simulink model "SCUTERacing_Model"  (R2020a)
settings: Solver=ode23tb  StartTime=0.0  StopTime=60  RelTol=5e-3
model workspace (MAT data in the model file):
  DLCXref = [0 8 9.5 18 34 34.5 45 50 60]
  DLCYref = [0 0 -4.5 -4 -3.75 1.5 0.5 0 0]
  VEH.Mass = 330
  VEH.StaticNormalFrontLoad.FR = 74.25
  VEH.StaticNormalFrontLoad.FL = 74.25
  VEH.StaticNormalRearLoad.RR = 90.75
  VEH.StaticNormalRearLoad.RL = 90.75
  VEH.WheelBase = 1.54
  VEH.FrontAxlePositionfromCG = 0.847
  VEH.RearAxlePositionfromCG = 0.693
  VEH.HeightCG = 0.283
  VEH.FrontalArea = 2.11
  VEH.DragCoefficient = 0.33
  VEH.NumberOfWheelsPerAxle = 2
  VEH.Thread.FR = 1.705
  VEH.Thread.RR = 1.705
  VEH.PitchMomentInertia = 206
  VEH.RollMomentInertia = 206.613792
  VEH.YawMomentInertia = 206.613792
  VEH.SteeringRatio = 5.2
  VEH.TrackWidth = 1.2
  VEH.SprungMass = 290
  VEH.InitialLongPosition = 0
  VEH.InitialLatPosition = 0
  VEH.InitialVertPosition = 0
  VEH.InitialRollAngle = 0
  VEH.InitialPitchAngle = 0
  VEH.InitialYawAngle = 0
  VEH.InitialLongVel = 0
  VEH.InitialLatVel = 0
  VEH.InitialVertVel = 0
  VEH.InitialRollRate = 0
  VEH.InitialPitchRate = 0
  VEH.InitialYawRate = 0
  extRef = 0.01
  mot.max_trq = 135
  mot.max_pwr = 38
  mot.spd = [370 739.166666667 1108.33333333 1477.5 1846.66666667 2215.83333333 2585 2954.16666667 3323.33333333 3692.5 4061.66666667 4430.83333333 4800]
  mot.trq = [135 135 135 135 135 135 130 125 120 90 80 72 65]
  mot.trq_cp = [120 112.169118269 105.297671501 99.2195136541 93.8047673037 88.9504392721 84.5738066939 80.6076640699 76.9968477689 73.6956545886 70.6658970819 90.4670202838 85.9436692696 81.8511135901 78.1306084269 74.7336254518 71.6197243914 68.7549354157]
  mot.mapL.spdindex = [100 200 300 400 500 600 700 800 900 1000 1100 1200 1300 1400 1500 1600 1700 1800 1900 2000 2100 2200 2300 2400 2500 2600 2700 2800 2900 3000 3100 3200 3300 3400 3500 3600 3700 3800 3900 4000 4100 4200 4300 4400 4500 4600 4700 4800]
  mot.mapL.trqindex = [7.5 15 22.5 30 37.5 45 52.5 60 67.5 75 82.5 90 97.5 105 112.5]
  mot.mapL.eff = [23.367031145 28.3093935 27.900833785 23.94351616 23.192960095 18.35774057 20.08454116 17.944414665 15.71176136 14.08332132 13.191387315 11.66605693 ... (720 elements, 15x48)]
  mot.mapR.spdindex = [100 200 300 400 500 600 700 800 900 1000 1100 1200 1300 1400 1500 1600 1700 1800 1900 2000 2100 2200 2300 2400 2500 2600 2700 2800 2900 3000 3100 3200 3300 3400 3500 3600 3700 3800 3900 4000 4100 4200 4300 4400 4500 4600 4700 4800]
  mot.mapR.trqindex = [7.5 15 22.5 30 37.5 45 52.5 60 67.5 75 82.5 90 97.5 105 112.5]
  mot.mapR.eff = [28.48167539 36.0807345 35.29712042 34.7163836 33.02727304 31.53442549 31.60094145 28.55014096 26.94374363 27.02005929 24.78971019 24.19758491 ... (720 elements, 15x48)]
undefined symbols (not defined in the file or in its folder): Batt, h, Right
libraries: simulink x6, vehdynlibscenariocommon x4, sim3dlib x2, vehdynlibdriver x1, autolibshared x1, vehdynlibviscommon x1
(part 1 of 2)
settings Model: SimulationMode=accelerator  Creator=Administrator  LastModifiedBy=Administrator
settings SolverCC: ZeroCrossAlgorithm=Adaptive
settings DataIOCC: DSMLogging=off
settings DebuggingCC: IgnoredZcDiagnostic=none

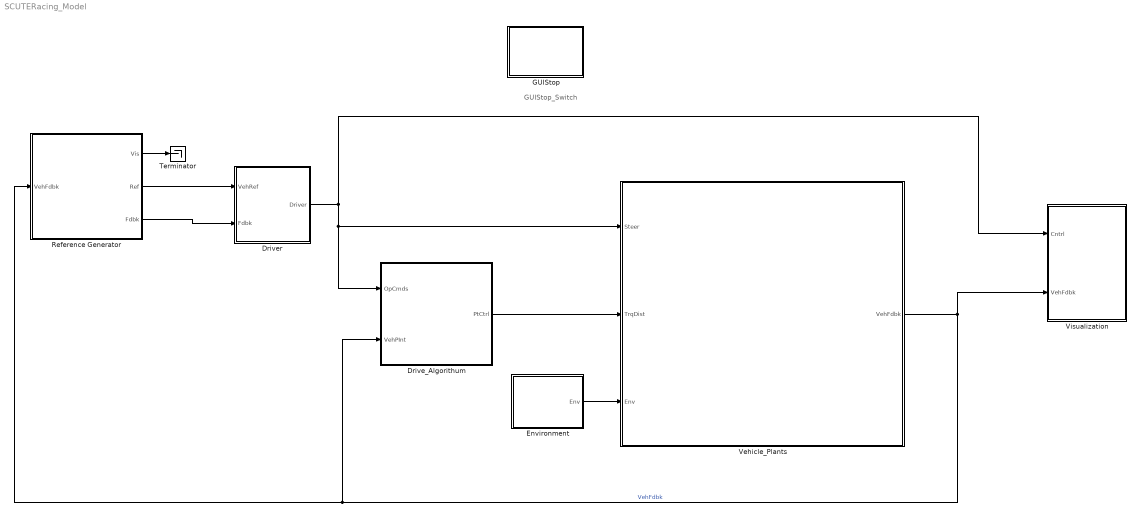
== system SCUTERacing_Model ==
  note: GUIStop_Switch
  Drive_Algorithum : Subsystem
      mask Display: image("Model_Pictures/SystemControllers.png")
  Driver : Subsystem
      mask Display: image("Model_Pictures/LongitudinalDriver.png")
  Environment : Subsystem
  GUIStop : Subsystem
  Reference Generator : Subsystem  Variant=on  VariantControl=Variant1
  Terminator : Terminator
  Vehicle_Plants : Subsystem
      mask Display: image("Model_Pictures/PassengerVehicle.png")
  Visualization : Subsystem
  wires:
  Reference Generator/1(" Vis") -> Terminator/1
  Reference Generator/2(" Ref") -> Driver/1(VehRef)
  Reference Generator/3(" Fdbk") -> Driver/2(Fdbk)
  Drive_Algorithum/1(PtCtrl) -> Vehicle_Plants/2(TrqDist)
  Vehicle_Plants/1(VehFdbk) -> Visualization/2(VehFdbk), Reference Generator/1("VehFdbk "), Drive_Algorithum/2(VehPInt)  "VehFdbk"
  Driver/1(Driver) -> Drive_Algorithum/1(OpCmds), Vehicle_Plants/1(Steer), Visualization/1(Cntrl)
  Environment/1(Env) -> Vehicle_Plants/3(Env)

== system SCUTERacing_Model/Drive_Algorithum ==
  OpCmds : Inport
  VehPInt : Inport  Port=2
  Algorithum : Subsystem
  outport_Module : Subsystem
  PtCtrl : Outport
  wires:
  Algorithum/1(BrakeCmd) -> outport_Module/1(BrakeCmd)
  VehPInt/1 -> Algorithum/2(VehPInt)
  Algorithum/2(MotCmd_L) -> outport_Module/2(MotCmd_L)
  Algorithum/3(MotCmd_R) -> outport_Module/3(MotCmd_R)
  outport_Module/1(OpCmd) -> PtCtrl/1
  OpCmds/1 -> Algorithum/1(OpCmds)

== system SCUTERacing_Model/Driver ==
  VehRef : Inport
  Fdbk : Inport  Port=2
  Bus Creator : BusCreator  Inputs=3
  Bus Selector : BusSelector  OutputSignals=Chassis.xdot,Chassis.Y,Chassis.ydot,Chassis.psi,Chassis.r
  Bus Selector1 : BusSelector  OutputSignals=LngRef,LtrlRef,AccelZero
  Constant : Constant  Value=0
  Dead Zone : DeadZone  ZeroCross=off  SaturateOnIntegerOverflow=on
  Dead Zone1 : DeadZone  LowerValue=-1e-2  UpperValue=1e-2  ZeroCross=off  SaturateOnIntegerOverflow=on
  Ground : Ground
  Predictive Driver : vehdynlibdriver/Predictive Driver  extAccelOvr=off  extDecelOvr=off  extAccelHld=off  extDecelHld=off  extAccelZero=off  extDecelZero=off  extSteerOvr=off  extSteerHld=off  extSteerZero=off  cntrlType=PI  shftType=None  velUnits=m/s  gearOut=off  steerOut=off  Kp=10  Ki=5  Kff=.1  Kg=0  VehVelVec=[0 100]  KffVec=[.1 .1]  KpVec=[10 10]  KiVec=[5 5]  KgVec=[0 0]  vnom=35  Kaw=1  tauerr=.01  a=VEH.FrontAxlePositionfromCG  b=VEH.RearAxlePositionfromCG  m=VEH.Mass  I=VEH.YawMomentInertia  Cy_f=11459  Cy_r=11459  theta=30*pi/180  Ksteer=18  tau=0.03  L=1.0  Kpt=3000  aR=200  bR=2.5  cR=.5  g=9.81  GearInit=0  tShift=.1  pdlVec=[0.1 0.4 0.5 0.9]  upShftTbl=[-1 12.9375 26.4375 39.9375 51.18749999999999 62.4375 72.84375 83.25;-1 16.3125 29.8125 43.3125 54.5624 65.8125 76.78125 87.75;-1 19.6875 33.1875 46.68749999999999 57.9375 69.1875 80.71875 92.25;-1 33 52.5 77.25 100.5 138.75 161.875 185]  dwnShftTbl=[-1 12.9375 26.4375 39.9375 51.18749999999999 62.4375 72.84375 83.25;-1 16.3125 29.8125 43.3125 54.5624 65.8125 76.78125 87.75;-1 19.6875 33.1875 46.68749999999999 57.9375 69.1875 80.71875 92.25;-1 33 52.5 77.25 100.5 138.75 161.875 185]  tClutch=.5  tRev=.5  tPark=120  aMode=2  UpGearVec="[0  1  2  3  4  5  6  7]"  DownGearVec="[1  2  3  4  5  6  7  8]"
      settings: SourceProductBaseCode=VE
  Switch : Switch  Criteria=u2 > Threshold
  Terminator1 : Terminator
  Wheel Angle Limit * Steer Ratio : Gain  Gain=20*pi/180*5.2
  Driver : Outport  VectorParamsAs1DForOutWhenUnconnected=off
  wires:
  Fdbk/1 -> Bus Selector/1
  Bus Creator/1 -> Driver/1
  Bus Selector1/1 -> Predictive Driver/1  "<LngRef>"
  Bus Selector/3 -> Predictive Driver/6  "<ydot>"
  Bus Selector/4 -> Predictive Driver/7  "<psi>"
  Switch/1 -> Bus Creator/2  "Accel"
  Bus Selector/1 -> Dead Zone/1  "<xdot>"
  Predictive Driver/3 -> Switch/3  "AccelCmd"
  Bus Selector1/2 -> Predictive Driver/2  "<LtrlRef>"
  Dead Zone/1 -> Predictive Driver/4
  Bus Selector/2 -> Predictive Driver/5  "<Y>"
  Dead Zone1/1 -> Wheel Angle Limit * Steer Ratio/1
  Predictive Driver/4 -> Bus Creator/3  "Brake"
  Wheel Angle Limit * Steer Ratio/1 -> Bus Creator/1  "Steer"
  Predictive Driver/1 -> Terminator1/1
  Bus Selector1/3 -> Switch/2  "<AccelZero>"
  Bus Selector/5 -> Predictive Driver/8  "<r>"
  Constant/1 -> Switch/1
  Ground/1 -> Predictive Driver/3
  VehRef/1 -> Bus Selector1/1
  Predictive Driver/2 -> Dead Zone1/1  "SteerCmd"

== system SCUTERacing_Model/Environment ==
  note: 注释：
      | 1）输入：
      | 1.Temp:环境温度
      | 2.Wind:模拟风速（x,y,z三个坐标）
      | 3.Gnd: a.G
      | b. friction:摩擦力（FL：前左轮；FR：前右轮；RL：后左轮；FL:后右轮）
      |
      | 2）输出：
      | 环境条件 Env ：
      | Temp：温度
      | Wind：风向
      | Gnd：地面参数
  Bus Creator : BusCreator  Inputs=4
  Bus Creator1 : BusCreator  Inputs=3
  Bus Creator2 : BusCreator  Inputs=4
  Bus Creator3 : BusCreator  Inputs=2
  Constant1 : Constant  Value=zeros(4,1)
  Constant3 : Constant  Value=0
  Constant4 : Constant  Value=0
  Constant5 : Constant  Value=0
  Constant6 : Constant  Value=300
  Demux : Demux
  Demux1 : Demux
  Friction : Constant  Value=ones(4,1).*1
  Vector Concatenate : Concatenate  NumInputs=3
  Env : Outport  VectorParamsAs1DForOutWhenUnconnected=off
  wires:
  Friction/1 -> Demux1/1
  Demux1/4 -> Bus Creator2/4  "mu_RR"
  Demux1/3 -> Bus Creator2/3  "mu_RL"
  Demux/1 -> Bus Creator/1  "G_FL_z"
  Vector Concatenate/1 -> Bus Creator1/2  "Wind"
  Demux1/1 -> Bus Creator2/1  "mu_FL"
  Constant1/1 -> Demux/1
  Bus Creator1/1 -> Env/1
  Bus Creator3/1 -> Bus Creator1/3  "Gnd"
  Demux1/2 -> Bus Creator2/2  "mu_FR"
  Constant6/1 -> Bus Creator1/1  "Temp"
  Demux/4 -> Bus Creator/4  "G_RR_z"
  Constant4/1 -> Vector Concatenate/2  "Y"
  Demux/2 -> Bus Creator/2  "G_FR_z"
  Demux/3 -> Bus Creator/3  "G_RL_z"
  Constant3/1 -> Vector Concatenate/1  "X"
  Constant5/1 -> Vector Concatenate/3  "Z"
  Bus Creator/1 -> Bus Creator3/1  "z"
  Bus Creator2/1 -> Bus Creator3/2  "mu"

== system SCUTERacing_Model/GUIStop ==
  S-Function : S-Function  FunctionName=StopFlag  SFunctionDeploymentMode=off  EnableBusSupport=off
  Stop Simulation : Stop
  wires:
  S-Function/1 -> Stop Simulation/1

== system SCUTERacing_Model/Reference Generator ==
  "VehFdbk " : Inport
  Constant Radius : Subsystem  VariantControl=RG==4  mask{t_start=0, xdot_r=120, xdotUnit=mph, R=22.5, turnDirMask=Right, ay_max=0.5, ay_stop=off, Parameter6=2}
      mask prompts: t_start "Maneuver start time, t_start [s]:"; xdot_r "Longitudinal velocity reference, xdot_r:"; xdotUnit "Longitudinal velocity reference units, xdotUnit []:"; R "Radius value, R [m]:"; turnDirMask "Turn direction"; ay_max "Lateral acceleration absolute threshold, ay_max [g]:"; ay_stop "Stop simulation at lateral acceleration threshold"
      mask TypeOptions xdotUnit: Longitudinal Velocity Reference/Input Units/Unit
      mask TypeOptions R: Constant Radius/Value
      mask TypeOptions turnDirMask: Constant Radius/turnDirMask
  Increasing Steer : Subsystem  VariantControl=RG==1
  Longitual_increasing : Subsystem  VariantControl=RG==0
  RealRunData : Subsystem  VariantControl=RG==5
  Sine with Dwell : Subsystem  VariantControl=RG==3
  Swept Sine : Subsystem  VariantControl=RG==2
  " Vis" : Outport  VectorParamsAs1DForOutWhenUnconnected=off
  " Ref" : Outport  Port=2  VectorParamsAs1DForOutWhenUnconnected=off
  " Fdbk" : Outport  Port=3  VectorParamsAs1DForOutWhenUnconnected=off

== system SCUTERacing_Model/Vehicle_Plants ==
  Steer : Inport
  TrqDist : Inport  Port=2
  Env : Inport  Port=3
  Bus Creator : BusCreator  Inputs=6
  Elect_Plant : Subsystem
  Steer_Sys : Subsystem
  Vehicle_Body : Subsystem
  VehFdbk : Outport
  wires:
  [MotSpd_L] -> Elect_Plant/5(Veh_L)
  Env/1 -> Elect_Plant/3(Env), Vehicle_Body/1(Env)
  Elect_Plant/1(ElecFdbk) -> Bus Creator/1, [ElecFdbk]  "ElecFdbk"
  [MotSpd_R] -> Elect_Plant/4(Veh_R)
  Vehicle_Body/3(MotSpd_L) -> Bus Creator/5, [MotSpd_L]  "MotSpd_L"
  Steer_Sys/1(DriveLine) -> Bus Creator/2, [DriveLine]  "DriveLine"
  Vehicle_Body/2(Wheels) -> Bus Creator/4, [Wheels]  "Wheels"
  Vehicle_Body/4(MotSpd_R) -> Bus Creator/6, [MotSpd_R]  "MotSpd_R"
  TrqDist/1 -> Elect_Plant/2(Ctrl_L), Steer_Sys/1(Contrl), Elect_Plant/1(Ctrl_R)
  Vehicle_Body/1(Chassis) -> Bus Creator/3  "Chassis"
  [DriveLine] -> Vehicle_Body/2(DriveLine)
  [ElecFdbk] -> Steer_Sys/3(ElecFdbk)
  [Wheels] -> Steer_Sys/4(Wheels)
  Steer/1 -> Steer_Sys/2(Steer)
  Bus Creator/1 -> VehFdbk/1

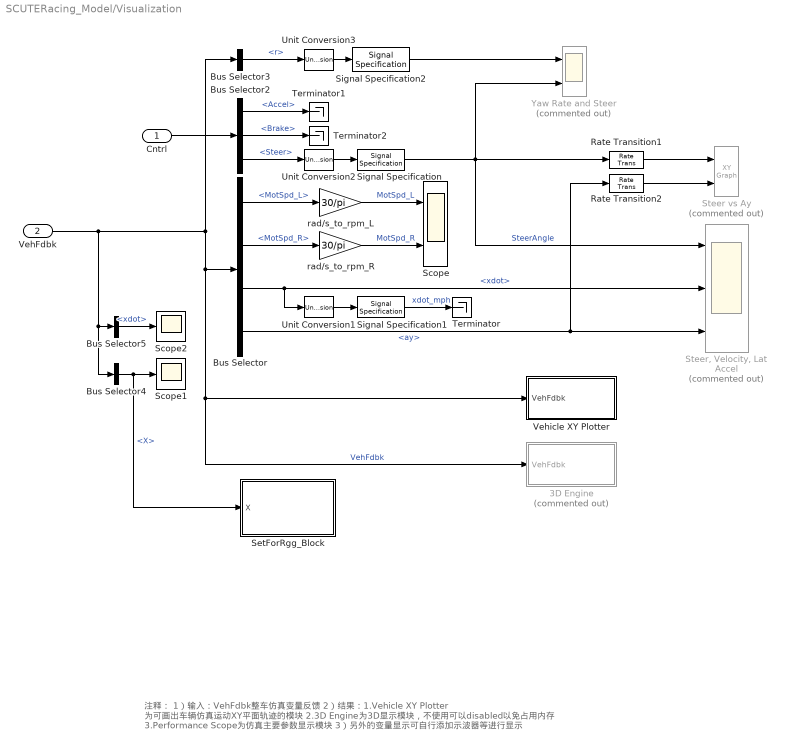
== system SCUTERacing_Model/Visualization ==
  note: 注释：
      | 1）输入：VehFdbk整车仿真变量反馈
      | 2）结果：1.Vehicle XY Plotter 为可画出车辆仿真运动XY平面轨迹的模块
      | 2.3D Engine为3D显示模块，不使用可以disabled以免占用内存
      | 3.Performance Scope为仿真主要参数显示模块
      | 3）另外的变量显示可自行添加示波器等进行显示
  Cntrl : Inport
  VehFdbk : Inport  Port=2
  3D Engine : Subsystem  Commented=on  Variant=on  VariantControlMode=Label  LabelModeActiveChoice=0  mask(3D Engine){engine3D=Disabled, SceneDesc=Straight road, dt3D=.03}
      mask prompts: engine3D "3D Engine"; SceneDesc "Scene Description:"; dt3D "Engine frame rate, dt3D [s]:"
      mask help: This subsystem contains the interface blocks which permit the display of the vehicle in 3D virtual environment. Enable it to view the simulation progress, disable it to inhibit the display.
      mask init:
      | switch get_param(gcb,'engine3D')
      |     case 'Disabled'
      |         set_param(gcb,'OverrideUsingVariant','0')
      |     case 'Enabled'
      |        set_param(gcb,'OverrideUsingVariant','1')
      |     otherwise
      |        set_param(gcb,'OverrideUsingVariant','0')
      | end
      settings: AttributesFormatString=%<engine3D>
      mask Help: eval('vdynblkshelp(''vdynblksscenecameraray'')');
      mask TypeOptions engine3D: Enabled | Disabled
      mask Callback engine3D:
      | switch get_param(gcb,'engine3D')
      |     case 'Disabled'
      |         set_param(gcb,'OverrideUsingVariant','0')
      |     case 'Enabled'
      |        set_param(gcb,'OverrideUsingVariant','1')
      |     otherwise
      |        set_param(gcb,'OverrideUsingVariant','0')
      | end
      mask TypeOptions SceneDesc:
      | 3D Engine/Simulation 3D Engine
      | 1/SceneDesc
      mask Display: disp('3D Engine')
  Bus Selector : BusSelector  OutputSignals=MotSpd_L,MotSpd_R,Chassis.xdot,Chassis.ay
  Bus Selector2 : BusSelector  OutputSignals=Accel,Brake,Steer
  Bus Selector3 : BusSelector  OutputSignals=Chassis.r
  Bus Selector4 : BusSelector  OutputSignals=Chassis.X
  Bus Selector5 : BusSelector  OutputSignals=Chassis.xdot
  Rate Transition1 : RateTransition  OutPortSampleTime=.1
  Rate Transition2 : RateTransition  OutPortSampleTime=.1
  Scope : Scope  NumInputPorts=2
  Scope1 : Scope
  Scope2 : Scope
  SetForRgg_Block : Subsystem
  Signal Specification : SignalSpecification  Unit=deg
  Signal Specification1 : SignalSpecification  Unit=mph
  Signal Specification2 : SignalSpecification  Unit=deg/s
  Steer vs Ay : simulink/Sinks/XY Graph  Commented=on  xmin=-300  xmax=300  ymin=-1.5  ymax=1.5  st=.1
  "Steer, Velocity, Lat Accel" : Scope  Commented=on  NumInputPorts=3
  Terminator : Terminator
  Terminator1 : Terminator
  Terminator2 : Terminator
  Unit Conversion1 : UnitConversion
  Unit Conversion2 : UnitConversion
  Unit Conversion3 : UnitConversion
  Vehicle XY Plotter : Subsystem  mask(Vehicle XY Plotter){a=VEH.FrontAxlePositionfromCG, b=VEH.RearAxlePositionfromCG, w=VEH.TrackWidth, bufferSize=1024, pltDT=.1}
      mask prompts: a "Distance to front axle from CG, a [m]:"; b "Distance to rear axle from CG, b [m]:"; w "Track width, w [m]:"; bufferSize "Path buffer sampe size, bufferSize []:"; pltDT "Plot update rate, pltDT [s]:"
      mask help: This block will display a MATLAB figure which indicates the vehicle path, current position and heading velocity.
      mask TypeOptions a: Vehicle XY Plotter/a
      mask TypeOptions b: Vehicle XY Plotter/b
      mask TypeOptions w: Vehicle XY Plotter/w
      mask TypeOptions bufferSize: Vehicle XY Plotter/bufferSize
  Yaw Rate and Steer : Scope  Commented=on  NumInputPorts=2
  rad/s_to_rpm_L : Gain  Gain=30/pi
  rad/s_to_rpm_R : Gain  Gain=30/pi
  wires:
  Unit Conversion2/1 -> Signal Specification/1
  Signal Specification/1 -> Yaw Rate and Steer/2, Rate Transition1/1, "Steer, Velocity, Lat Accel"/1  "SteerAngle"
  Bus Selector2/1 -> Terminator1/1  "<Accel>"
  Bus Selector3/1 -> Unit Conversion3/1  "<r>"
  Signal Specification2/1 -> Yaw Rate and Steer/1
  Cntrl/1 -> Bus Selector2/1
  Rate Transition2/1 -> Steer vs Ay/2
  Rate Transition1/1 -> Steer vs Ay/1
  rad/s_to_rpm_L/1 -> Scope/1  "MotSpd_L"
  Bus Selector4/1 -> SetForRgg_Block/1(X), Scope1/1  "<X>"
  Bus Selector/2 -> rad/s_to_rpm_R/1  "<MotSpd_R>"
  Bus Selector/1 -> rad/s_to_rpm_L/1  "<MotSpd_L>"
  Bus Selector2/3 -> Unit Conversion2/1  "<Steer>"
  Unit Conversion1/1 -> Signal Specification1/1
  VehFdbk/1 -> Bus Selector5/1, Bus Selector4/1, Bus Selector/1, Vehicle XY Plotter/1(VehFdbk), 3D Engine/1(VehFdbk), Bus Selector3/1  "VehFdbk"
  Bus Selector2/2 -> Terminator2/1  "<Brake>"
  Unit Conversion3/1 -> Signal Specification2/1
  Bus Selector5/1 -> Scope2/1  "<xdot>"
  Signal Specification1/1 -> Terminator/1  "xdot_mph"
  Bus Selector/3 -> Unit Conversion1/1, "Steer, Velocity, Lat Accel"/2  "<xdot>"
  rad/s_to_rpm_R/1 -> Scope/2  "MotSpd_R"
  Bus Selector/4 -> Rate Transition2/1, "Steer, Velocity, Lat Accel"/3  "<ay>"

== system SCUTERacing_Model/Drive_Algorithum/Algorithum ==
  OpCmds : Inport
  VehPInt : Inport  Port=2
  Algorithum_VariantModel : Subsystem  Variant=on
  Mux : Mux
  "Power Management " : Subsystem
  Subsystem : Subsystem
  inportModule : Subsystem
  BrakeCmd : Outport
  MotCmd_L : Outport  Port=2
  MotCmd_R : Outport  Port=3
  wires:
  Mux/1 -> BrakeCmd/1
  OpCmds/1 -> inportModule/1(OpCmds)
  VehPInt/1 -> inportModule/2(VehPInt)
  inportModule/1(AccCmd) -> Subsystem/2(AccCmd), Algorithum_VariantModel/1(AccCmd)
  inportModule/10(WhlAng) -> Algorithum_VariantModel/10(WhlAng)
  inportModule/11(Spd) -> Algorithum_VariantModel/11(Spd)
  inportModule/8(Steer) -> Algorithum_VariantModel/8(Steer)
  inportModule/9(YawRate) -> Algorithum_VariantModel/9(YawRate)
  inportModule/2(MotSpd_L) -> [MotSpd_L], Subsystem/3(MotSpd_L), Algorithum_VariantModel/2(MotSpd_L)
  inportModule/3(MotSpd_R) -> [MotSpd_R], Subsystem/1(MotSpd_R), Algorithum_VariantModel/3(MotSpd_R)
  inportModule/4(VehSpd(km/h)) -> Algorithum_VariantModel/4(VehSpd)
  inportModule/5(DecCmd) -> Algorithum_VariantModel/5(DecCmd)
  inportModule/6(MotPwr_L) -> Algorithum_VariantModel/6(MotPwr_L)
  inportModule/7(MotPwr_R) -> Algorithum_VariantModel/7(MotPwr_R)
  inportModule/12(BattSOC) -> Algorithum_VariantModel/12(BattSOC)
  Subsystem/1(MotTrqCmd_L) -> Algorithum_VariantModel/13(MotTrqCmd_L)
  Subsystem/2(MotTrqCmd_R) -> Algorithum_VariantModel/14(MotTrqCmd_R)
  Algorithum_VariantModel/3(Fric_Brake) -> Mux/4, Mux/3, Mux/2, Mux/1
  Algorithum_VariantModel/1(Final_MotTrqReq_L) -> "Power Management "/1(MotTrqReq_L)
  Algorithum_VariantModel/2(Final_MotTrqReq_R) -> "Power Management "/2(MotTrqReq_R)
  inportModule/13(BattVolt) -> [BattVolt]
  [MotSpd_R] -> "Power Management "/4(MotSpd_R)
  [MotSpd_L] -> "Power Management "/3(MotSpd_L)
  [BattVolt] -> "Power Management "/5(BattV)
  "Power Management "/2(MotTrqReqAllow_R) -> MotCmd_R/1
  "Power Management "/1(MotTrqReqAllow_L) -> MotCmd_L/1

== system SCUTERacing_Model/Drive_Algorithum/outport_Module ==
  BrakeCmd : Inport
  MotCmd_L : Inport  Port=2
  MotCmd_R : Inport  Port=3
  Bus Creator : BusCreator  Inputs=3
  Memory : Memory
  Rate Transition : RateTransition  Deterministic=off
  Rate Transition1 : RateTransition  Deterministic=off
  Rate Transition2 : RateTransition  Deterministic=off
  OpCmd : Outport
  wires:
  BrakeCmd/1 -> Rate Transition/1
  MotCmd_L/1 -> Rate Transition1/1
  MotCmd_R/1 -> Rate Transition2/1
  Rate Transition/1 -> Memory/1
  Rate Transition1/1 -> Bus Creator/2  "MotCmd_L"
  Rate Transition2/1 -> Bus Creator/3  "MotCmd_R"
  Bus Creator/1 -> OpCmd/1
  Memory/1 -> Bus Creator/1  "BrakeCmd"

== system SCUTERacing_Model/Reference Generator/Constant Radius ==
  "VehFdbk " : Inport
  Bus Assignment : BusAssignment  AssignedSignals=Chassis.Y
  Bus Creator : BusCreator  Inputs=3
  Bus Creator1 : BusCreator  Inputs=5
  Bus Selector1 : BusSelector  OutputSignals=Chassis.ay
  Bus Selector2 : BusSelector  OutputSignals=Chassis.X,Chassis.Y,Chassis.psi,Chassis.Z
  Constant : Constant  Value=0
  Constant Radius : Subsystem  mask{Value=R, turnDirMask=Right}
      mask prompts: Value "Simulink:blkprm_prompts:ConstConstValue"; turnDirMask "Turn direction"
      mask TypeOptions Value: R/Value
      mask TypeOptions turnDirMask: Left | Right
      mask DialogControl Value Prompt: Constant value:
  Constant1 : Constant  Value=0  OutDataTypeStr=boolean
  Constant2 : Constant  Value=0
  Constant3 : Constant  Value=0  OutDataTypeStr=boolean
  Longitudinal Velocity Reference : Subsystem
  Signal Copy : SignalConversion  OverrideOpt=off
  Signal Specification : SignalSpecification  Unit=m
  ay Stop : vehdynlibscenariocommon/Slowly Increasing Steer/ay Stop  SystemSampleTime=-1  Latency=0  AutoFrameSizeCalculation=off
      settings: SourceProductBaseCode=VE
  " Vis" : Outport  VectorParamsAs1DForOutWhenUnconnected=off
  " Ref" : Outport  Port=2  VectorParamsAs1DForOutWhenUnconnected=off
  " Fdbk" : Outport  Port=3  VectorParamsAs1DForOutWhenUnconnected=off
  wires:
  Constant3/1 -> Bus Creator1/3  "EnblSteerCmd"
  Constant2/1 -> Bus Creator1/4  "SteerOvrCmd"
  Longitudinal Velocity Reference/1(xdot) -> Bus Creator1/1  "LngRef"
  Signal Specification/1 -> Bus Creator1/2  "LtrlRef"
  Bus Creator1/1 -> " Ref"/1
  Constant1/1 -> Bus Creator1/5  "AccelZero"
  Constant/1 -> Signal Specification/1
  Constant Radius/1(yRef) -> Bus Assignment/2  "LatRef"
  Bus Assignment/1 -> " Fdbk"/1
  Signal Copy/1 -> Bus Creator/3  "ZRef"
  Bus Creator/1 -> " Vis"/1
  Bus Selector2/4 -> Signal Copy/1  "<Z>"
  Constant Radius/3(YRef) -> Bus Creator/2  "YRef"
  "VehFdbk "/1 -> Bus Selector2/1, Bus Assignment/1, Bus Selector1/1
  Bus Selector2/2 -> Constant Radius/2(YVeh)  "<Y>"
  Bus Selector2/3 -> Constant Radius/3(psiVeh)  "<psi>"
  Bus Selector2/1 -> Constant Radius/1(XVeh)  "<X>"
  Constant Radius/2(XRef) -> Bus Creator/1  "XRef"
  Bus Selector1/1 -> ay Stop/1  "<ay>"

== system SCUTERacing_Model/Reference Generator/Increasing Steer ==
  "VehFdbk " : Inport
  Bus Creator : BusCreator  Inputs=3
  Ground : Ground
  Ground1 : Ground
  Ground2 : Ground
  Increasing Steer : vehdynlibscenariocommon/Slowly Increasing Steer  VariantControl=1  t_start=0  xdot_r=35  xdotUnit=mph  omega_hw=13.5  theta_max=90  t_stop=60  ay_max=0.5  ay_stop=on  aMode=2
      settings: SourceProductBaseCode=VE
  " Vis" : Outport  VectorParamsAs1DForOutWhenUnconnected=off
  " Ref" : Outport  Port=2  VectorParamsAs1DForOutWhenUnconnected=off
  " Fdbk" : Outport  Port=3  VectorParamsAs1DForOutWhenUnconnected=off
  wires:
  Ground/1 -> Bus Creator/1  "XRef"
  Ground1/1 -> Bus Creator/2  "YRef"
  Ground2/1 -> Bus Creator/3  "ZRef"
  Increasing Steer/1 -> " Ref"/1  "LtrlRef"
  Bus Creator/1 -> " Vis"/1
  "VehFdbk "/1 -> Increasing Steer/1, " Fdbk"/1

== system SCUTERacing_Model/Reference Generator/Longitual_increasing ==
  "VehFdbk " : Inport
  Bus Creator : BusCreator  Inputs=3
  Ground : Ground
  Ground1 : Ground
  Ground2 : Ground
  Ramp : simulink/Sources/Ramp  slope=100  start=0  InitialOutput=0  VectorParams1D=off
  Saturation : Saturate  UpperLimit=80
      settings: LockScale=on
  Signal Specification1 : SignalSpecification  Unit=m/s
  Signal Specification2 : SignalSpecification  Unit=mph
  Unit Conversion1 : UnitConversion
  " Vis" : Outport
  " Ref" : Outport  Port=2
  " Fdbk" : Outport  Port=3
  wires:
  "VehFdbk "/1 -> " Fdbk"/1
  Ground/1 -> " Vis"/1
  Ramp/1 -> Saturation/1
  Unit Conversion1/1 -> Signal Specification1/1
  Bus Creator/1 -> " Ref"/1
  Signal Specification1/1 -> Bus Creator/1  "LngRef"
  Ground1/1 -> Bus Creator/2  "LtrlRef"
  Ground2/1 -> Bus Creator/3  "AccelZero"
  Saturation/1 -> Signal Specification2/1
  Signal Specification2/1 -> Unit Conversion1/1  "Km/h"

== system SCUTERacing_Model/Reference Generator/RealRunData ==
  "VehFdbk " : Inport
  Bus Creator : BusCreator  Inputs=3
  Drive Cycle Source : autolibshared/Drive Cycle Source  cycleVar=.mat, .xls, .xlsx or .txt file  fileVar=C:\Users\Administrator\Desktop\新建文件夹 (3)\Scutracing\SCUTRacing\Eracing2020\SCUTRacing_EF20SimulinkProject\mFile\xdotref.mat  tfinal="2273  seconds"  cycleRepeat=off  outAccPort=off  outGearPort=off  gearList=No gear data  t_wot1=5  xdot_woto=0  xdot_wot1=30  t_wot2=20  xdot_wot2=0  t_wotend=30  srcUnit=km/h  outUnit=mph  srcAccUnit=m/s/s  outAccUnit=m/s^2  dt=0  aMode=1  faultOption=off  velBnd=2  velBndUnit=mph  inUnit=m/s  timeBnd=1  failOption=off  stopSim=off  maxFaultCnt=10  maxFaultTime=2  maxTotFaultTime=15  traceOption=off  dtTrace=1  traceWindow=10  lastDCname=Custom Data Set  lastOutUnit=mph  lastDT=0  lastTB=1  lastSB=2  forceCalcBound=off
      settings: AttributesFormatString=耐久跑动3圈数据 (%<tfinal>)  SourceProductBaseCode=PW
  Ground : Ground
  Ground1 : Ground
  Ground2 : Ground
  SetForRgg_Block2 : Subsystem  Commented=on
  " Vis" : Outport
  " Ref" : Outport  Port=2
  " Fdbk" : Outport  Port=3
  wires:
  "VehFdbk "/1 -> " Fdbk"/1
  Ground/1 -> " Vis"/1
  Bus Creator/1 -> " Ref"/1
  Drive Cycle Source/1 -> SetForRgg_Block2/1(LngRef), Bus Creator/1  "LngRef"
  Ground1/1 -> Bus Creator/2  "LtrlRef"
  Ground2/1 -> Bus Creator/3  "AccelZero"

== system SCUTERacing_Model/Reference Generator/Sine with Dwell ==
  "VehFdbk " : Inport
  Bus Creator : BusCreator  Inputs=3
  Ground : Ground
  Ground1 : Ground
  Ground2 : Ground
  Sine With Dwell : vehdynlibscenariocommon/Sine With Dwell  VariantControl=3  t_start=0  xdot_r=30  xdotUnit=mph  steerF=7  steerA=90  tdwell=0.5  steerDir=off  aMode=2
      settings: SourceProductBaseCode=VE
  " Vis" : Outport  VectorParamsAs1DForOutWhenUnconnected=off
  " Ref" : Outport  Port=2  VectorParamsAs1DForOutWhenUnconnected=off
  " Fdbk" : Outport  Port=3  VectorParamsAs1DForOutWhenUnconnected=off
  wires:
  Ground/1 -> Bus Creator/1  "XRef"
  Ground1/1 -> Bus Creator/2  "YRef"
  Ground2/1 -> Bus Creator/3  "ZRef"
  Bus Creator/1 -> " Vis"/1
  "VehFdbk "/1 -> Sine With Dwell/1, " Fdbk"/1
  Sine With Dwell/1 -> " Ref"/1

== system SCUTERacing_Model/Reference Generator/Swept Sine ==
  "VehFdbk " : Inport
  Bus Creator : BusCreator  Inputs=3
  Ground : Ground
  Ground1 : Ground
  Ground2 : Ground
  Swept Sine : vehdynlibscenariocommon/Swept Sine Reference Generator  VariantControl=2  t_start=1  xdot_r=35  xdotUnit=mph  theta_hw=90  theta_hw_final=0.7  t_sweep=30  aMode=2
      settings: SourceProductBaseCode=VE
  " Vis" : Outport  VectorParamsAs1DForOutWhenUnconnected=off
  " Ref" : Outport  Port=2  VectorParamsAs1DForOutWhenUnconnected=off
  " Fdbk" : Outport  Port=3  VectorParamsAs1DForOutWhenUnconnected=off
  wires:
  Ground/1 -> Bus Creator/1  "XRef"
  Ground1/1 -> Bus Creator/2  "YRef"
  Ground2/1 -> Bus Creator/3  "ZRef"
  Bus Creator/1 -> " Vis"/1
  Swept Sine/1 -> " Ref"/1
  "VehFdbk "/1 -> Swept Sine/1, " Fdbk"/1

== system SCUTERacing_Model/Vehicle_Plants/Elect_Plant ==
  Ctrl_R : Inport
  Ctrl_L : Inport  Port=2
  Env : Inport  Port=3
  Veh_R : Inport  Port=4
  Veh_L : Inport  Port=5
  EP_InportModule : Subsystem
  EP_Module : Subsystem
  EP_OutportModule : Subsystem
  ElecFdbk : Outport
  wires:
  Veh_L/1 -> EP_InportModule/5(Veh_L)
  Ctrl_R/1 -> EP_InportModule/1(Ctrl_R)
  Ctrl_L/1 -> EP_InportModule/2(Ctrl_L)
  Env/1 -> EP_InportModule/3(Env)
  Veh_R/1 -> EP_InportModule/4(Veh_R)
  EP_Module/1(MotTrq_L) -> EP_OutportModule/1(MotTrq_L)
  EP_Module/2(MotPwr_L) -> EP_OutportModule/2(MotPwr_L)
  EP_Module/3(MotTrq_R) -> EP_OutportModule/3(MotTrq_R)
  EP_Module/4(BattCrnt) -> EP_OutportModule/4(BattCrnt)
  EP_Module/5(MotPwr_R) -> EP_OutportModule/5(MotPwr_R)
  EP_Module/6(BattSOC) -> EP_OutportModule/6(BattSOC)
  EP_Module/7(BattV) -> EP_OutportModule/7(BattVolt)
  EP_Module/8(BattPwr) -> EP_OutportModule/8(BattPwr)
  EP_OutportModule/1(ElecFdbk) -> ElecFdbk/1
  EP_InportModule/5(AmbTmp) -> EP_Module/5(BattTemp)
  EP_InportModule/3(MotTrqCmd_R) -> EP_Module/3(MotTrqCmd_R)
  EP_InportModule/4(MotSpd_R) -> EP_Module/4(MotSpd_R)
  EP_InportModule/2(MotSpd_L) -> EP_Module/2(MotSpd_L)
  EP_InportModule/1(MotTrqCmd_L) -> EP_Module/1(MotTrqCmd_L)

== system SCUTERacing_Model/Vehicle_Plants/Steer_Sys ==
  Contrl : Inport
  Steer : Inport  Port=2
  ElecFdbk : Inport  Port=3
  Wheels : Inport  Port=4
  SS_InportModule : Subsystem
  SS_Module : ModelReference  ModelNameDialog=Driveline.slx  ModelReferenceVersion=1.213
  SS_Outport : Subsystem
  DriveLine : Outport
  wires:
  Contrl/1 -> SS_InportModule/1(Contrl)
  SS_InportModule/1(Steer) -> SS_Module/1
  SS_InportModule/2(MotTrq_L) -> SS_Module/2
  SS_InportModule/3(MotTrq_R) -> SS_Module/3
  SS_InportModule/4(PrsCmd) -> SS_Module/4
  SS_InportModule/5(Omega) -> SS_Module/5
  Steer/1 -> SS_InportModule/2(SteerCmd)
  Wheels/1 -> SS_InportModule/4(Wheels)
  ElecFdbk/1 -> SS_InportModule/3(ElecFdbk)
  SS_Module/1 -> SS_Outport/1(WhlAng)
  SS_Module/2 -> SS_Outport/2(AxlTrq)
  SS_Module/3 -> SS_Outport/3(BrkPrs)
  SS_Outport/1(DriverLine) -> DriveLine/1

== system SCUTERacing_Model/Vehicle_Plants/Vehicle_Body ==
  Env : Inport
  DriveLine : Inport  Port=2
  PassVeh7DOF : ModelReference  ModelNameDialog=PassVeh7DOF.slx  ModelReferenceVersion=1.132
      settings: PortSchema="{\"entries\":[{\"content\":{\"sides\":[{\"content\":{\"connectorIds\":[\"In1\",\"In2\",\"In3\",\"In4\",\"In5\",\"In6\"]},\"type\":\"ConnectorPlacement.EquallySpacedRectSide\",\"uuid\":\"c13e2a57-6282-469b-bf8c-5ef2cf5e4289\"},{\"content\":{\"connectorIds\":[\"Out1\",\"Out2\",\"Out3\",\"Out4\",\"Out5\",\"Out6\",\"Out7\",\"Out8\",\"Out9\",\"Out10\",\"Out11\",\"Out12\",\"Out13\",\"Out16\",\"Out14\",\"Out17\",\"Out15\",\"Out18\",\"Out19\",\"Out20\"],\"side\":\"RIGHT\"},\"type\":\"ConnectorPlacement.EquallySpacedRectSide\",\"uuid\":\"5967b75c-68c3-49cd-a0fa-646ea2f0b31f\"},{\"content\":{\"connectorIds\":[],\"side\":\"TOP\"},\"type\":\"ConnectorPlacement.EquallySpacedRectSide\",\"uuid\":\"e6c409ca-5b37-47ae-8d18-8691f7fcce92\"}]},\"type\":\"ConnectorPlacement.EquallySpacedConnector\",\"uuid\":\"965b2ed5-89d3-4a02-963e-cde21217ac56\"}],\"packageUris\":[\"http://schema.mathworks.com/mf0/Connector/19700101\"],\"version\":\"1.0\"}"
  VB_InportModule : Subsystem
  VB_OutportModule : Subsystem
  Chassis : Outport
  Wheels : Outport  Port=2
  MotSpd_L : Outport  Port=3
  MotSpd_R : Outport  Port=4
  wires:
  Env/1 -> VB_InportModule/1(Env)
  DriveLine/1 -> VB_InportModule/2(DriveLine)
  PassVeh7DOF/1 -> VB_OutportModule/1(xdot)
  PassVeh7DOF/2 -> VB_OutportModule/2(ydot)
  PassVeh7DOF/3 -> VB_OutportModule/3(X)
  PassVeh7DOF/4 -> VB_OutportModule/4(Y)
  PassVeh7DOF/5 -> VB_OutportModule/5(Z)
  PassVeh7DOF/6 -> VB_OutportModule/6(Xdot)
  PassVeh7DOF/7 -> VB_OutportModule/7(Ydot)
  PassVeh7DOF/8 -> VB_OutportModule/8(phi)
  PassVeh7DOF/9 -> VB_OutportModule/9(theta)
  PassVeh7DOF/10 -> VB_OutportModule/10(psi)
  PassVeh7DOF/11 -> VB_OutportModule/11(p)
  PassVeh7DOF/12 -> VB_OutportModule/12(q)
  PassVeh7DOF/13 -> VB_OutportModule/13(r)
  VB_OutportModule/1(Chassis) -> Chassis/1
  VB_OutportModule/2(Wheels) -> Wheels/1
  VB_OutportModule/3(MotSpd_L) -> MotSpd_L/1
  VB_OutportModule/4(MotSpd_R) -> MotSpd_R/1
  VB_InportModule/1(AxleTrq) -> PassVeh7DOF/1
  VB_InportModule/2(BrkPrs) -> PassVeh7DOF/2
  VB_InportModule/3(Wind) -> PassVeh7DOF/3
  VB_InportModule/4(WhlAng) -> PassVeh7DOF/4
  VB_InportModule/5(GND) -> PassVeh7DOF/5
  VB_InportModule/6(mu) -> PassVeh7DOF/6
  PassVeh7DOF/16 -> VB_OutportModule/14(ay)
  PassVeh7DOF/14 -> VB_OutportModule/15(kappa)
  PassVeh7DOF/17 -> VB_OutportModule/16(zAxle)
  PassVeh7DOF/15 -> VB_OutportModule/17(omega)
  PassVeh7DOF/18 -> VB_OutportModule/18(ZHP)
  PassVeh7DOF/19 -> VB_OutportModule/19(XWheel)
  PassVeh7DOF/20 -> VB_OutportModule/20(YWheel)

== system SCUTERacing_Model/Visualization/3D Engine ==
  note: 1) Add Subsystem or Model blocks as valid variant choices.
      | 2) You cannot connect blocks at this level. At simulation, connectivity is automatically
      | determined, based on the active variant and port name matching.
  VehFdbk : Inport
  3D Engine : Subsystem  VariantControl=1
  3D Engine Disabled : Subsystem  VariantControl=0

== system SCUTERacing_Model/Visualization/SetForRgg_Block ==
  X : Inport
  Compare To Constant : simulink/Logic and Bit Operations/Compare To Constant  relop=>=  const=75  OutDataTypeStr=boolean
  Logical Operator : Logic  AllPortsSameDT=off  OutDataTypeStr=boolean
  Set_For_Rgg : Constant  OutDataTypeStr=boolean
  Stop Simulation : Stop
  To Workspace : ToWorkspace  VariableName=Flag  SaveFormat=Structure  SampleTime=-1
      settings: Save2DSignal=2-D array (concatenate along first dimension)
  wires:
  Compare To Constant/1 -> Logical Operator/1
  X/1 -> Compare To Constant/1
  Logical Operator/1 -> To Workspace/1, Stop Simulation/1
  Set_For_Rgg/1 -> Logical Operator/2

== system SCUTERacing_Model/Visualization/Vehicle XY Plotter ==
  VehFdbk : Inport
  Bus Selector1 : BusSelector  OutputSignals=Chassis.phi,Chassis.theta,Chassis.psi  OutputAsBus=on
  Bus Selector2 : BusSelector  OutputSignals=DriveLine.WhlAng  OutputAsBus=on
  Bus Selector3 : BusSelector  OutputSignals=Chassis.X,Chassis.Y,Chassis.Z  OutputAsBus=on
  Bus Selector4 : BusSelector  OutputSignals=Chassis.Xdot,Chassis.Ydot  OutputAsBus=on
  Bus to Vector{,1..3} (4 alike) : BusToVector
  Ground : Ground
  Ground1 : Ground
  Rate Transition{1..2,5..6} (4 alike) : RateTransition  OutPortSampleTime=pltDT
  Vector Concatenate : Concatenate
  Vehicle XY Plotter : vehdynlibviscommon/Vehicle XY Plotter  bufferSize=bufferSize  w=w  a=a  b=b  figBorder=10
      settings: SourceProductBaseCode=VE
  wires:
  Bus to Vector2/1 -> Rate Transition1/1  "InertCGDisp"
  Rate Transition5/1 -> Vehicle XY Plotter/1
  Bus Selector4/1 -> Bus to Vector1/1
  Rate Transition1/1 -> Vehicle XY Plotter/2
  Rate Transition6/1 -> Vehicle XY Plotter/3
  Vector Concatenate/1 -> Rate Transition6/1  "InertCGVel"
  Bus Selector1/1 -> Bus to Vector2/1
  Bus to Vector/1 -> Rate Transition5/1  "InertCGDisp"
  Bus Selector3/1 -> Bus to Vector/1
  Bus to Vector1/1 -> Vector Concatenate/1
  Ground/1 -> Vector Concatenate/2
  Bus to Vector3/1 -> Rate Transition2/1
  Bus Selector2/1 -> Bus to Vector3/1
  VehFdbk/1 -> Bus Selector1/1, Bus Selector2/1, Bus Selector4/1, Bus Selector3/1
  Rate Transition2/1 -> Vehicle XY Plotter/4
  Ground1/1 -> Vehicle XY Plotter/5

== system SCUTERacing_Model/Drive_Algorithum/Algorithum/Algorithum_VariantModel ==
  AccCmd : Inport
  MotSpd_L : Inport  Port=2
  MotSpd_R : Inport  Port=3
  VehSpd : Inport  Port=4
  DecCmd : Inport  Port=5
  MotPwr_L : Inport  Port=6
  MotPwr_R : Inport  Port=7
  Steer : Inport  Port=8
  YawRate : Inport  Port=9
  WhlAng : Inport  Port=10
  Spd : Inport  Port=11
  BattSOC : Inport  Port=12
  MotTrqCmd_L : Inport  Port=13
  MotTrqCmd_R : Inport  Port=14
  BERS : ModelReference  ModelNameDialog=BERS.slx  VariantControl=AV==1  ModelReferenceVersion=1.3
  EDS : ModelReference  DisableCoverage=on  ModelNameDialog=EDS.slx  VariantControl=AV==2  ModelReferenceVersion=1.7
  EF20Algo : ModelReference  ModelNameDialog=EF20Algo.slx  VariantControl=AV==3  ModelReferenceVersion=1.15
  TCS : ModelReference  ModelNameDialog=TCS.slx  VariantControl=AV==0  ModelReferenceVersion=1.14
  Final_MotTrqReq_L : Outport
  Final_MotTrqReq_R : Outport  Port=2
  Fric_Brake : Outport  Port=3

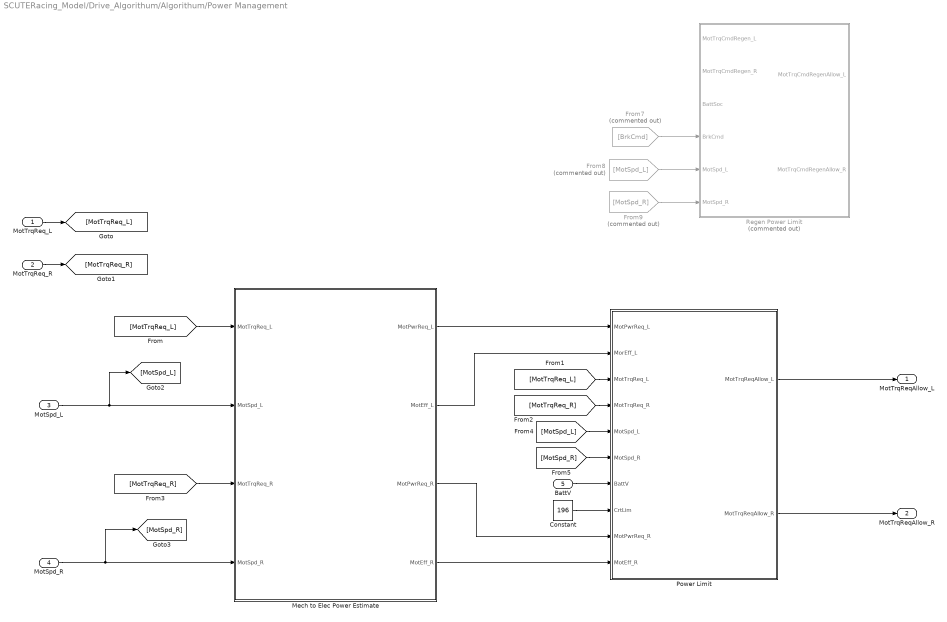
== system SCUTERacing_Model/Drive_Algorithum/Algorithum/Power Management  ==
  MotTrqReq_L : Inport
  MotTrqReq_R : Inport  Port=2
  MotSpd_L : Inport  Port=3
  MotSpd_R : Inport  Port=4
  BattV : Inport  Port=5
  Constant : Constant  Value=196
  From7 : From  Commented=on  GotoTag=BrkCmd
  From8 : From  Commented=on  GotoTag=MotSpd_L
  From9 : From  Commented=on  GotoTag=MotSpd_R
  Mech to Elec Power Estimate : Subsystem
  Power Limit : Subsystem
  Regen Power Limit : Subsystem  Commented=on
  MotTrqReqAllow_L : Outport  VectorParamsAs1DForOutWhenUnconnected=off
  MotTrqReqAllow_R : Outport  Port=2  VectorParamsAs1DForOutWhenUnconnected=off
  wires:
  MotSpd_L/1 -> [MotSpd_L], Mech to Elec Power Estimate/2(MotSpd_L)
  MotSpd_R/1 -> [MotSpd_R], Mech to Elec Power Estimate/4(MotSpd_R)
  MotTrqReq_L/1 -> [MotTrqReq_L]
  MotTrqReq_R/1 -> [MotTrqReq_R]
  [MotTrqReq_L] -> Power Limit/3(MotTrqReq_L)
  [MotTrqReq_R] -> Power Limit/4(MotTrqReq_R)
  [MotSpd_L] -> Power Limit/5(MotSpd_L)
  [MotSpd_R] -> Power Limit/6(MotSpd_R)
  BattV/1 -> Power Limit/7(BattV)
  Constant/1 -> Power Limit/8(CrtLim)
  From8/1 -> Regen Power Limit/5(MotSpd_L)
  From9/1 -> Regen Power Limit/6(MotSpd_R)
  From7/1 -> Regen Power Limit/4(BrkCmd)
  [MotTrqReq_L] -> Mech to Elec Power Estimate/1(MotTrqReq_L)
  [MotTrqReq_R] -> Mech to Elec Power Estimate/3(MotTrqReq_R)
  Mech to Elec Power Estimate/1(MotPwrReq_L) -> Power Limit/1(MotPwrReq_L)
  Mech to Elec Power Estimate/3(MotPwrReq_R) -> Power Limit/9(MotPwrReq_R)
  Mech to Elec Power Estimate/2(MotEff_L) -> Power Limit/2(MorEff_L)
  Mech to Elec Power Estimate/4(MotEff_R) -> Power Limit/10(MotEff_R)
  Power Limit/1(MotTrqReqAllow_L) -> MotTrqReqAllow_L/1
  Power Limit/2(MotTrqReqAllow_R) -> MotTrqReqAllow_R/1

== system SCUTERacing_Model/Drive_Algorithum/Algorithum/Subsystem ==
  MotSpd_R : Inport
  AccCmd : Inport  Port=2
  MotSpd_L : Inport  Port=3
  Max Motor Trq vs. Spd Curve : Lookup_n-D  NumberOfTableDimensions=1  BreakpointsForDimension1=mot.spd  Table=mot.trq  UseLastTableValue=on  InternalRulePriority=Speed  OutDataTypeStr=Inherit: Inherit from 'Table data'  RndMeth=Simplest  InputSameDT=on
  Max Motor Trq vs. Spd Curve1 : Lookup_n-D  NumberOfTableDimensions=1  BreakpointsForDimension1=mot.spd  Table=mot.trq  UseLastTableValue=on  InternalRulePriority=Speed  OutDataTypeStr=Inherit: Inherit from 'Table data'  RndMeth=Simplest  InputSameDT=on
  Product1 : Product
  Product3 : Product
  MotTrqCmd_L : Outport
  MotTrqCmd_R : Outport  Port=2
  wires:
  AccCmd/1 -> Product1/1, Product3/2
  Product3/1 -> MotTrqCmd_L/1
  Product1/1 -> MotTrqCmd_R/1
  Max Motor Trq vs. Spd Curve1/1 -> Product3/1
  Max Motor Trq vs. Spd Curve/1 -> Product1/2
  MotSpd_L/1 -> Max Motor Trq vs. Spd Curve/1
  MotSpd_R/1 -> Max Motor Trq vs. Spd Curve1/1

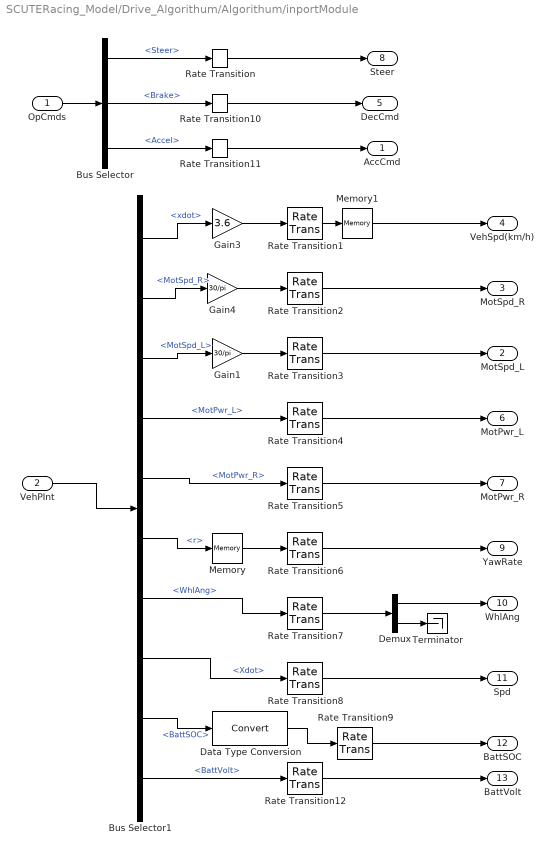
== system SCUTERacing_Model/Drive_Algorithum/Algorithum/inportModule ==
  OpCmds : Inport
  VehPInt : Inport  Port=2
  Bus Selector : BusSelector  OutputSignals=Steer,Brake,Accel
  Bus Selector1 : BusSelector  OutputSignals=Chassis.xdot,MotSpd_R,MotSpd_L,ElecFdbk.MotPwr_L,ElecFdbk.MotPwr_R,Chassis.r,DriveLine.WhlAng,Chassis.Xdot,ElecFdbk.BattSOC,ElecFdbk.BattVolt
  Data Type Conversion : DataTypeConversion
  Demux : Demux  Outputs=2
  Gain1 : Gain  Gain=30/pi
  Gain3 : Gain  Gain=3.6
  Gain4 : Gain  Gain=30/pi
  Memory : Memory
  Memory1 : Memory
  Rate Transition{,1..6,10..11} (9 alike) : RateTransition  Deterministic=off
  Rate Transition{7..9,12} (4 alike) : RateTransition
  Terminator : Terminator
  AccCmd : Outport
  MotSpd_L : Outport  Port=2
  MotSpd_R : Outport  Port=3
  VehSpd(km/h) : Outport  Port=4
  DecCmd : Outport  Port=5
  MotPwr_L : Outport  Port=6
  MotPwr_R : Outport  Port=7
  Steer : Outport  Port=8
  YawRate : Outport  Port=9
  WhlAng : Outport  Port=10
  Spd : Outport  Port=11
  BattSOC : Outport  Port=12
  BattVolt : Outport  Port=13
  wires:
  Bus Selector/2 -> Rate Transition10/1  "<Brake>"
  OpCmds/1 -> Bus Selector/1
  Bus Selector/1 -> Rate Transition/1  "<Steer>"
  VehPInt/1 -> Bus Selector1/1
  Rate Transition1/1 -> Memory1/1
  Bus Selector1/1 -> Gain3/1  "<xdot>"
  Bus Selector1/2 -> Gain4/1  "<MotSpd_R>"
  Bus Selector1/3 -> Gain1/1  "<MotSpd_L>"
  Bus Selector1/4 -> Rate Transition4/1  "<MotPwr_L>"
  Bus Selector1/5 -> Rate Transition5/1  "<MotPwr_R>"
  Bus Selector1/6 -> Memory/1  "<r>"
  Bus Selector1/7 -> Rate Transition7/1  "<WhlAng>"
  Bus Selector1/8 -> Rate Transition8/1  "<Xdot>"
  Rate Transition2/1 -> MotSpd_R/1
  Rate Transition3/1 -> MotSpd_L/1
  Rate Transition4/1 -> MotPwr_L/1
  Rate Transition5/1 -> MotPwr_R/1
  Rate Transition6/1 -> YawRate/1
  Rate Transition8/1 -> Spd/1
  Rate Transition9/1 -> BattSOC/1
  Bus Selector1/9 -> Data Type Conversion/1  "<BattSOC>"
  Bus Selector/3 -> Rate Transition11/1  "<Accel>"
  Rate Transition10/1 -> DecCmd/1
  Rate Transition11/1 -> AccCmd/1
  Rate Transition/1 -> Steer/1
  Rate Transition7/1 -> Demux/1
  Demux/1 -> WhlAng/1
  Demux/2 -> Terminator/1
  Memory/1 -> Rate Transition6/1
  Gain3/1 -> Rate Transition1/1
  Gain4/1 -> Rate Transition2/1
  Gain1/1 -> Rate Transition3/1
  Memory1/1 -> VehSpd(km/h)/1
  Bus Selector1/10 -> Rate Transition12/1  "<BattVolt>"
  Rate Transition12/1 -> BattVolt/1
  Data Type Conversion/1 -> Rate Transition9/1

== system SCUTERacing_Model/Reference Generator/Constant Radius/Constant Radius ==
  XVeh : Inport
  YVeh : Inport  Port=2
  psiVeh : Inport  Port=3
  Constant5 : Constant
  Demux : Demux  Outputs=3
  Demux1 : Demux  Outputs=3
  Ground1 : Ground
  IC : InitialCondition  Value=0
  MATLAB Function : MATLAB Function  TreatAsAtomicUnit=on
  Mux : Mux  Inputs=3
  Mux1 : Mux  Inputs=3
  R : Constant  Value=Value
  Signal Specification1 : SignalSpecification  Unit=m
  Signal Specification2 : SignalSpecification  Unit=m
  Signal Specification3 : SignalSpecification  Unit=m
  Switch : Switch  Criteria=u2 > Threshold
  Terminator1 : Terminator
  Unit Delay : UnitDelay  SampleTime=-1  HasFrameUpgradeWarning=on
  yRef : Outport  VectorParamsAs1DForOutWhenUnconnected=off
  XRef : Outport  Port=2  VectorParamsAs1DForOutWhenUnconnected=off
  YRef : Outport  Port=3  VectorParamsAs1DForOutWhenUnconnected=off
  wires:
  MATLAB Function/2(VehRef) -> Demux1/1
  Signal Specification3/1 -> yRef/1
  MATLAB Function/1(yRef) -> Signal Specification3/1
  Signal Specification2/1 -> XRef/1
  Signal Specification1/1 -> YRef/1
  Demux1/1 -> Signal Specification2/1
  Demux1/2 -> Signal Specification1/1
  Demux1/3 -> Terminator1/1
  psiVeh/1 -> Mux1/3
  R/1 -> MATLAB Function/1(Rref)
  Unit Delay/1 -> Switch/1
  Mux1/1 -> Switch/3
  IC/1 -> Switch/2
  Ground1/1 -> Mux/3
  Switch/1 -> Unit Delay/1, Demux/1
  Demux/1 -> MATLAB Function/3(Xo)
  Demux/3 -> MATLAB Function/5(psio)
  XVeh/1 -> Mux1/1, Mux/1
  Demux/2 -> MATLAB Function/4(Yo)
  YVeh/1 -> Mux1/2, Mux/2
  Constant5/1 -> IC/1
  Mux/1 -> MATLAB Function/2(InertCGDisp)

== system SCUTERacing_Model/Reference Generator/Constant Radius/Longitudinal Velocity Reference ==
  Input Units : SignalSpecification  Unit=mph
  Ramp1 : simulink/Sources/Ramp  slope=100  start=t_start  InitialOutput=0
  Saturation1 : Saturate  UpperLimit=xdot_r  LowerLimit=0  ZeroCross=off
  Signal Specification1 : SignalSpecification  Unit=m/s
  Unit Conversion1 : UnitConversion
  xdot : Outport  VectorParamsAs1DForOutWhenUnconnected=off
  wires:
  Unit Conversion1/1 -> Signal Specification1/1
  Signal Specification1/1 -> xdot/1
  Saturation1/1 -> Input Units/1
  Ramp1/1 -> Saturation1/1
  Input Units/1 -> Unit Conversion1/1

== system SCUTERacing_Model/Reference Generator/RealRunData/SetForRgg_Block2 ==
  LngRef : Inport
  Compare To Constant : simulink/Logic and Bit Operations/Compare To Constant  relop=<  const=0.0001  OutDataTypeStr=boolean
  Logical Operator : Logic  AllPortsSameDT=off  OutDataTypeStr=boolean
  Set_For_Rgg : Constant  OutDataTypeStr=boolean
  Stop Simulation : Stop
  To Workspace : ToWorkspace  VariableName=Flag_nj  SaveFormat=Structure  SampleTime=-1
      settings: Save2DSignal=2-D array (concatenate along first dimension)
  wires:
  Set_For_Rgg/1 -> Logical Operator/2
  Logical Operator/1 -> To Workspace/1, Stop Simulation/1
  Compare To Constant/1 -> Logical Operator/1
  LngRef/1 -> Compare To Constant/1

== system SCUTERacing_Model/Vehicle_Plants/Elect_Plant/EP_InportModule ==
  Ctrl_R : Inport
  Ctrl_L : Inport  Port=2
  Env : Inport  Port=3
  Veh_R : Inport  Port=4
  Veh_L : Inport  Port=5
  Bus Selector : BusSelector  OutputSignals=MotCmd_R
  Bus Selector1 : BusSelector  OutputSignals=MotCmd_L
  Bus Selector2 : BusSelector  OutputSignals=Temp
  Rate Transition : RateTransition  Deterministic=off
  Rate Transition{1..4} (4 alike) : RateTransition
  MotTrqCmd_L : Outport
  MotSpd_L : Outport  Port=2
  MotTrqCmd_R : Outport  Port=3
  MotSpd_R : Outport  Port=4
  AmbTmp : Outport  Port=5
  wires:
  Bus Selector/1 -> Rate Transition/1  "<MotCmd_R>"
  Rate Transition/1 -> MotTrqCmd_R/1
  Ctrl_R/1 -> Bus Selector/1
  Ctrl_L/1 -> Bus Selector1/1
  Rate Transition1/1 -> MotTrqCmd_L/1
  Bus Selector1/1 -> Rate Transition1/1  "<MotCmd_L>"
  Bus Selector2/1 -> Rate Transition2/1  "<Temp>"
  Rate Transition2/1 -> AmbTmp/1
  Env/1 -> Bus Selector2/1
  Veh_L/1 -> Rate Transition4/1
  Veh_R/1 -> Rate Transition3/1
  Rate Transition4/1 -> MotSpd_L/1
  Rate Transition3/1 -> MotSpd_R/1

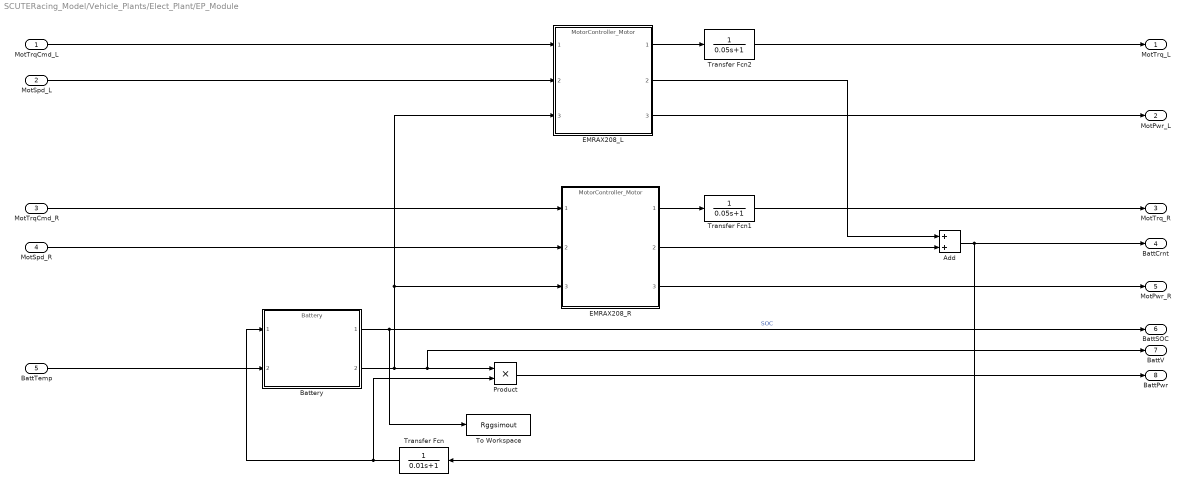
== system SCUTERacing_Model/Vehicle_Plants/Elect_Plant/EP_Module ==
  MotTrqCmd_L : Inport
  MotSpd_L : Inport  Port=2
  MotTrqCmd_R : Inport  Port=3
  MotSpd_R : Inport  Port=4
  BattTemp : Inport  Port=5
  Add : Sum
  Battery : ModelReference  ModelNameDialog=Battery.slx  ModelReferenceVersion=1.1
  EMRAX208_L : ModelReference  ModelNameDialog=MotorController_Motor.slx  ModelReferenceVersion=1.2
  EMRAX208_R : ModelReference  ModelNameDialog=MotorController_Motor.slx  ModelReferenceVersion=1.2
  Product : Product
  To Workspace : ToWorkspace  VariableName=Rggsimout  SaveFormat=Structure With Time  SampleTime=-1
  Transfer Fcn : TransferFcn  Denominator=[0.01 1]
  Transfer Fcn1 : TransferFcn  Denominator=[0.05 1]
  Transfer Fcn2 : TransferFcn  Denominator=[0.05 1]
  MotTrq_L : Outport
  MotPwr_L : Outport  Port=2
  MotTrq_R : Outport  Port=3
  BattCrnt : Outport  Port=4
  MotPwr_R : Outport  Port=5
  BattSOC : Outport  Port=6
  BattV : Outport  Port=7
  BattPwr : Outport  Port=8
  wires:
  Transfer Fcn/1 -> Product/2, Battery/1
  MotTrqCmd_L/1 -> EMRAX208_L/1
  EMRAX208_R/2 -> Add/2
  EMRAX208_R/3 -> MotPwr_R/1
  Add/1 -> BattCrnt/1, Transfer Fcn/1
  Battery/1 -> To Workspace/1, BattSOC/1  "SOC"
  EMRAX208_L/1 -> Transfer Fcn2/1
  Transfer Fcn2/1 -> MotTrq_L/1
  EMRAX208_L/2 -> Add/1
  MotSpd_R/1 -> EMRAX208_R/2
  Battery/2 -> EMRAX208_R/3, EMRAX208_L/3, BattV/1, Product/1
  EMRAX208_R/1 -> Transfer Fcn1/1
  EMRAX208_L/3 -> MotPwr_L/1
  Transfer Fcn1/1 -> MotTrq_R/1
  MotSpd_L/1 -> EMRAX208_L/2
  BattTemp/1 -> Battery/2
  MotTrqCmd_R/1 -> EMRAX208_R/1
  Product/1 -> BattPwr/1

== system SCUTERacing_Model/Vehicle_Plants/Elect_Plant/EP_OutportModule ==
  MotTrq_L : Inport
  MotPwr_L : Inport  Port=2
  MotTrq_R : Inport  Port=3
  BattCrnt : Inport  Port=4
  MotPwr_R : Inport  Port=5
  BattSOC : Inport  Port=6
  BattVolt : Inport  Port=7
  BattPwr : Inport  Port=8
  Bus Creator : BusCreator  Inputs=8
  ElecFdbk : Outport
  wires:
  MotPwr_R/1 -> Bus Creator/5  "MotPwr_R"
  BattCrnt/1 -> Bus Creator/4  "BattCrnt"
  Bus Creator/1 -> ElecFdbk/1
  MotTrq_R/1 -> Bus Creator/3  "MotTrq_R"
  MotPwr_L/1 -> Bus Creator/2  "MotPwr_L"
  BattVolt/1 -> Bus Creator/7  "BattVolt"
  MotTrq_L/1 -> Bus Creator/1  "MotTrq_L"
  BattPwr/1 -> Bus Creator/8  "BattPwr"
  BattSOC/1 -> Bus Creator/6  "BattSOC"

== system SCUTERacing_Model/Vehicle_Plants/Steer_Sys/SS_InportModule ==
  Contrl : Inport
  SteerCmd : Inport  Port=2
  ElecFdbk : Inport  Port=3
  Wheels : Inport  Port=4
  Bus Selector : BusSelector  OutputSignals=Steer
  Bus Selector1 : BusSelector  OutputSignals=MotTrq_L
  Bus Selector2 : BusSelector  OutputSignals=MotTrq_L
  Bus Selector3 : BusSelector  OutputSignals=BrakeCmd
  Bus Selector4 : BusSelector  OutputSignals=omega
  Steer : Outport
  MotTrq_L : Outport  Port=2
  MotTrq_R : Outport  Port=3
  PrsCmd : Outport  Port=4
  Omega : Outport  Port=5
  wires:
  Bus Selector/1 -> Steer/1  "<Steer>"
  SteerCmd/1 -> Bus Selector/1
  ElecFdbk/1 -> Bus Selector2/1, Bus Selector1/1
  Wheels/1 -> Bus Selector4/1
  Bus Selector4/1 -> Omega/1  "<omega>"
  Bus Selector3/1 -> PrsCmd/1  "<BrakeCmd>"
  Contrl/1 -> Bus Selector3/1
  Bus Selector1/1 -> MotTrq_L/1  "<MotTrq_L>"
  Bus Selector2/1 -> MotTrq_R/1  "<MotTrq_L>"

== system SCUTERacing_Model/Vehicle_Plants/Steer_Sys/SS_Outport ==
  WhlAng : Inport
  AxlTrq : Inport  Port=2
  BrkPrs : Inport  Port=3
  Bus Creator : BusCreator  Inputs=3
  DriverLine : Outport
  wires:
  AxlTrq/1 -> Bus Creator/2  "AxlTrq"
  WhlAng/1 -> Bus Creator/1  "WhlAng"
  BrkPrs/1 -> Bus Creator/3  "BrkPrs"
  Bus Creator/1 -> DriverLine/1

== system SCUTERacing_Model/Vehicle_Plants/Vehicle_Body/VB_InportModule ==
  Env : Inport
  DriveLine : Inport  Port=2
  Bus Selector : BusSelector  OutputSignals=Wind
  Bus Selector1 : BusSelector  OutputSignals=Gnd.z.G_FL_z,Gnd.z.G_FR_z,Gnd.z.G_RL_z,Gnd.z.G_RR_z
  Bus Selector2 : BusSelector  OutputSignals=Gnd.mu.mu_FL,Gnd.mu.mu_FR,Gnd.mu.mu_RL,Gnd.mu.mu_RR
  Bus Selector3 : BusSelector  OutputSignals=WhlAng,AxlTrq,BrkPrs
  Vector Concatenate : Concatenate  NumInputs=4
  Vector Concatenate1 : Concatenate  NumInputs=4
  AxleTrq : Outport
  BrkPrs : Outport  Port=2
  Wind : Outport  Port=3
  WhlAng : Outport  Port=4
  GND : Outport  Port=5
  mu : Outport  Port=6
  wires:
  Bus Selector/1 -> Wind/1  "<Wind>"
  Env/1 -> Bus Selector2/1, Bus Selector1/1, Bus Selector/1
  Bus Selector2/2 -> Vector Concatenate/2  "<mu_FR>"
  Vector Concatenate/1 -> mu/1
  Bus Selector2/1 -> Vector Concatenate/1  "<mu_FL>"
  Bus Selector1/1 -> Vector Concatenate1/1  "<G_FL_z>"
  Bus Selector1/2 -> Vector Concatenate1/2  "<G_FR_z>"
  Vector Concatenate1/1 -> GND/1
  DriveLine/1 -> Bus Selector3/1
  Bus Selector3/1 -> WhlAng/1  "<WhlAng>"
  Bus Selector3/2 -> AxleTrq/1  "<AxlTrq>"
  Bus Selector1/3 -> Vector Concatenate1/3  "<G_RL_z>"
  Bus Selector1/4 -> Vector Concatenate1/4  "<G_RR_z>"
  Bus Selector2/3 -> Vector Concatenate/3  "<mu_RL>"
  Bus Selector2/4 -> Vector Concatenate/4  "<mu_RR>"
  Bus Selector3/3 -> BrkPrs/1  "<BrkPrs>"

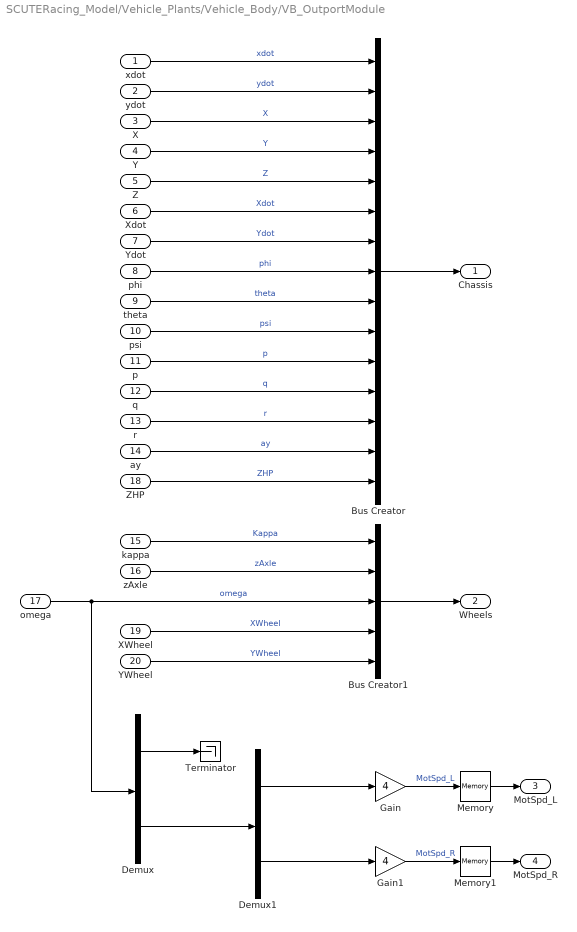
== system SCUTERacing_Model/Vehicle_Plants/Vehicle_Body/VB_OutportModule ==
  xdot : Inport
  ydot : Inport  Port=2
  X : Inport  Port=3
  Y : Inport  Port=4
  Z : Inport  Port=5
  Xdot : Inport  Port=6
  Ydot : Inport  Port=7
  phi : Inport  Port=8
  theta : Inport  Port=9
  psi : Inport  Port=10
  p : Inport  Port=11
  q : Inport  Port=12
  r : Inport  Port=13
  ay : Inport  Port=14
  kappa : Inport  Port=15
  zAxle : Inport  Port=16
  omega : Inport  Port=17
  ZHP : Inport  Port=18
  XWheel : Inport  Port=19
  YWheel : Inport  Port=20
  Bus Creator : BusCreator  Inputs=15
  Bus Creator1 : BusCreator  Inputs=5
  Demux : Demux  Outputs=2
  Demux1 : Demux  Outputs=2
  Gain : Gain  Gain=4
  Gain1 : Gain  Gain=4
  Memory : Memory
  Memory1 : Memory
  Terminator : Terminator
  Chassis : Outport
  Wheels : Outport  Port=2
  MotSpd_L : Outport  Port=3
  MotSpd_R : Outport  Port=4
  wires:
  Y/1 -> Bus Creator/4  "Y"
  Bus Creator/1 -> Chassis/1
  xdot/1 -> Bus Creator/1  "xdot"
  phi/1 -> Bus Creator/8  "phi"
  ydot/1 -> Bus Creator/2  "ydot"
  theta/1 -> Bus Creator/9  "theta"
  Xdot/1 -> Bus Creator/6  "Xdot"
  Z/1 -> Bus Creator/5  "Z"
  X/1 -> Bus Creator/3  "X"
  Ydot/1 -> Bus Creator/7  "Ydot"
  psi/1 -> Bus Creator/10  "psi"
  ay/1 -> Bus Creator/14  "ay"
  p/1 -> Bus Creator/11  "p"
  r/1 -> Bus Creator/13  "r"
  q/1 -> Bus Creator/12  "q"
  ZHP/1 -> Bus Creator/15  "ZHP"
  kappa/1 -> Bus Creator1/1  "Kappa"
  zAxle/1 -> Bus Creator1/2  "zAxle"
  omega/1 -> Demux/1, Bus Creator1/3  "omega"
  XWheel/1 -> Bus Creator1/4  "XWheel"
  YWheel/1 -> Bus Creator1/5  "YWheel"
  Demux/1 -> Terminator/1
  Demux/2 -> Demux1/1
  Demux1/1 -> Gain/1
  Demux1/2 -> Gain1/1
  Bus Creator1/1 -> Wheels/1
  Gain1/1 -> Memory1/1  "MotSpd_R"
  Gain/1 -> Memory/1  "MotSpd_L"
  Memory/1 -> MotSpd_L/1
  Memory1/1 -> MotSpd_R/1
